simulink model "Control_SMA"  (R2018a)
settings: Solver=VariableStepAuto  StartTime=0.0  StopTime=7  RelTol=1e-3
libraries: simulink x2, fuzblock x1
settings Model: Creator=Christyan  LastModifiedBy=Christyan

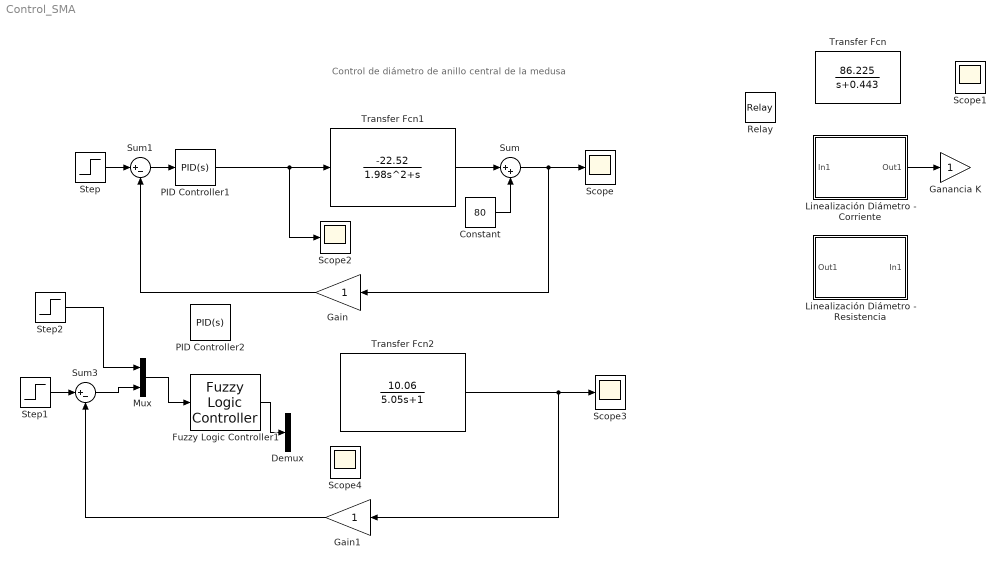
== system Control_SMA ==
  note: Control de diámetro de anillo central de la medusa
  Constant : Constant  Value=80
  Demux : Demux  Outputs=3
  Fuzzy Logic Controller1 : fuzblock/Fuzzy Logic  Controller  FIS='tipper.fis'  OutputSampleNumber=101  DataType=double  FuzzifiedInputs=off  RuleFiringStrengths=off  RuleOutputs=off  AggregatedOutputs=off  SimulateUsing=Interpreted execution  OutOfRangeInputValueMessage=warning  NoRuleFiredMessage=warning  EmptyOutputFuzzySetMessage=warning
  Gain : Gain
  Gain1 : Gain
  "Ganancia K " : Gain
  Linealización Diámetro - Corriente : Subsystem
  "Linealización Diámetro - Resistencia " : Subsystem
  Mux : Mux  Inputs=2
  PID Controller1 : simulink/Continuous/PID Controller  Controller=PID  TimeDomain=Continuous-time  SampleTime=-1  IntegratorMethod=Forward Euler  FilterMethod=Forward Euler  Form=Ideal  UseFilter=on  ControllerParametersSource=internal  P=-0.784515738735433  I=0.311823182176046  D=0.795359570303404  N=816.551119410098  InitialConditionSource=internal  InitialConditionForIntegrator=0  InitialConditionForFilter=0  ExternalReset=none  LimitOutput=off  UpperSaturationLimit=inf  LowerSaturationLimit=-inf  LinearizeAsGain=on  AntiWindupMode=none  Kb=1  TrackingMode=off  Kt=1  PParamMin=[]  PParamMax=[]  IParamMin=[]  IParamMax=[]  DParamMin=[]  DParamMax=[]  NParamMin=[]  NParamMax=[]  KbParamMin=[]  KbParamMax=[]  KtParamMin=[]  KtParamMax=[]  POutMin=[]  POutMax=[]  IOutMin=[]  IOutMax=[]  DOutMin=[]  DOutMax=[]  NOutMin=[]  NOutMax=[]  KbOutMin=[]  KbOutMax=[]  KtOutMin=[]  KtOutMax=[]  IntegratorOutMin=[]  IntegratorOutMax=[]  FilterOutMin=[]  FilterOutMax=[]  SumOutMin=[]  SumOutMax=[]  SumI1OutMin=[]  SumI1OutMax=[]  SumI2OutMin=[]  SumI2OutMax=[]  SumI3OutMin=[]  SumI3OutMax=[]  SumDOutMin=[]  SumDOutMax=[]  SaturationOutMin=[]  SaturationOutMax=[]  IntegratorContinuousStateAttributes=''  IntegratorStateMustResolveToSignalObject=off  IntegratorRTWStateStorageClass=Auto  FilterContinuousStateAttributes=''  FilterStateMustResolveToSignalObject=off  FilterRTWStateStorageClass=Auto  DifferentiatorICPrevScaledInput=0  DifferentiatorOutMin=[]  DifferentiatorOutMax=[]  FilterDiffOutCoefMin=[]  FilterDiffOutCoefMax=[]  SumDenOutMin=[]  SumDenOutMax=[]  SumNumOutMin=[]  SumNumOutMax=[]  ReciprocalOutMin=[]  ReciprocalOutMax=[]  DivideOutMin=[]  DivideOutMax=[]  TunerSelectOption=Transfer Function Based (PID Tuner App)
  PID Controller2 : simulink/Continuous/PID Controller  Controller=PID  TimeDomain=Continuous-time  SampleTime=-1  IntegratorMethod=Forward Euler  FilterMethod=Forward Euler  Form=Ideal  UseFilter=on  ControllerParametersSource=internal  P=1.04488712066562  I=0.670848029720148  D=0.0983891229337389  N=2.77143983520018  InitialConditionSource=internal  InitialConditionForIntegrator=0  InitialConditionForFilter=0  ExternalReset=none  LimitOutput=off  UpperSaturationLimit=inf  LowerSaturationLimit=-inf  LinearizeAsGain=on  AntiWindupMode=none  Kb=1  TrackingMode=off  Kt=1  PParamMin=[]  PParamMax=[]  IParamMin=[]  IParamMax=[]  DParamMin=[]  DParamMax=[]  NParamMin=[]  NParamMax=[]  KbParamMin=[]  KbParamMax=[]  KtParamMin=[]  KtParamMax=[]  POutMin=[]  POutMax=[]  IOutMin=[]  IOutMax=[]  DOutMin=[]  DOutMax=[]  NOutMin=[]  NOutMax=[]  KbOutMin=[]  KbOutMax=[]  KtOutMin=[]  KtOutMax=[]  IntegratorOutMin=[]  IntegratorOutMax=[]  FilterOutMin=[]  FilterOutMax=[]  SumOutMin=[]  SumOutMax=[]  SumI1OutMin=[]  SumI1OutMax=[]  SumI2OutMin=[]  SumI2OutMax=[]  SumI3OutMin=[]  SumI3OutMax=[]  SumDOutMin=[]  SumDOutMax=[]  SaturationOutMin=[]  SaturationOutMax=[]  IntegratorContinuousStateAttributes=''  IntegratorStateMustResolveToSignalObject=off  IntegratorRTWStateStorageClass=Auto  FilterContinuousStateAttributes=''  FilterStateMustResolveToSignalObject=off  FilterRTWStateStorageClass=Auto  DifferentiatorICPrevScaledInput=0  DifferentiatorOutMin=[]  DifferentiatorOutMax=[]  FilterDiffOutCoefMin=[]  FilterDiffOutCoefMax=[]  SumDenOutMin=[]  SumDenOutMax=[]  SumNumOutMin=[]  SumNumOutMax=[]  ReciprocalOutMin=[]  ReciprocalOutMax=[]  DivideOutMin=[]  DivideOutMax=[]  TunerSelectOption=Transfer Function Based (PID Tuner App)
  Relay : Relay
  Scope{,1..4} (5 alike) : Scope
  Step : Step  Time=0  After=45  SampleTime=0.33
  Step1 : Step  Time=0  After=5  SampleTime=0.33
  Step2 : Step  Time=0  After=5  SampleTime=0.33
  Sum : Sum  Inputs=|++
  Sum1 : Sum  Inputs=|+-
  Sum3 : Sum  Inputs=|+-
  Transfer Fcn : TransferFcn  Numerator=[86.225]  Denominator=[1 0.443]
  Transfer Fcn1 : TransferFcn  Numerator=[-22.52]  Denominator=[1.98 1 0]
  Transfer Fcn2 : TransferFcn  Numerator=[10.06]  Denominator=[5.05 1]
  wires:
  Linealización Diámetro - Corriente/1(Out1) -> "Ganancia K "/1
  Transfer Fcn1/1 -> Sum/1
  Constant/1 -> Sum/2
  Step/1 -> Sum1/1
  Gain/1 -> Sum1/2
  Sum/1 -> Gain/1, Scope/1
  Sum1/1 -> PID Controller1/1
  PID Controller1/1 -> Scope2/1, Transfer Fcn1/1
  Step1/1 -> Sum3/1
  Transfer Fcn2/1 -> Gain1/1, Scope3/1
  Gain1/1 -> Sum3/2
  Mux/1 -> Fuzzy Logic Controller1/1
  Fuzzy Logic Controller1/1 -> Demux/1
  Sum3/1 -> Mux/2
  Step2/1 -> Mux/1

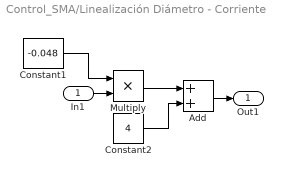
== system Control_SMA/Linealización Diámetro - Corriente ==
  In1 : Inport
  Add : Sum
  Constant1 : Constant  Value=-0.048
  Constant2 : Constant  Value=4
  Multiply : Product
  Out1 : Outport
  wires:
  Constant2/1 -> Add/2
  Constant1/1 -> Multiply/1
  Multiply/1 -> Add/1
  In1/1 -> Multiply/2
  Add/1 -> Out1/1

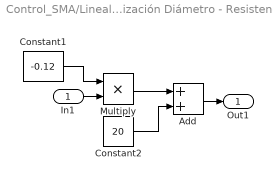
== system Control_SMA/Linealización Diámetro - Resistencia  ==
  In1 : Inport
  Add : Sum
  Constant1 : Constant  Value=-0.12
  Constant2 : Constant  Value=20
  Multiply : Product
  Out1 : Outport
  wires:
  Constant2/1 -> Add/2
  Constant1/1 -> Multiply/1
  Multiply/1 -> Add/1
  In1/1 -> Multiply/2
  Add/1 -> Out1/1
